simulink model "simple_relay_hysteresis"  (R2015a)
settings: Solver=ode45  StartTime=0.0  StopTime=tmax  RelTol=1e-3
values from neighbouring files (symbols this model uses):
  A = 5    [testing_simple_relay_hysteresis.m]
  b = 1    [testing_relay_plant_positive_feedback.m]    (also in testing_simple_relay_hysteresis.m = 1.5; testing_simple_relay_plant.m)
  d = 1    [testing_relay_plant_positive_feedback.m]    (also in testing_simple_relay_hysteresis.m = 2; testing_simple_relay_plant.m)
settings Model: Creator=ra428  LastModifiedBy=ra428

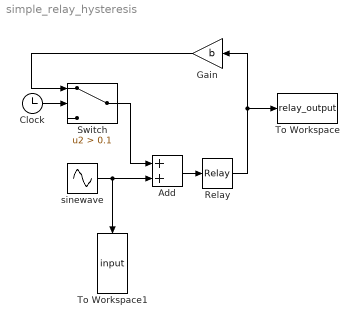
== system simple_relay_hysteresis ==
  Add : Sum
  Clock : Clock
  Gain : Gain  Gain=b
  Relay : Relay  OnSwitchValue=0  OffSwitchValue=0  OnOutputValue=d  OffOutputValue=-d
  Switch : Switch  Criteria=u2 > Threshold  Threshold=0.1
  To Workspace : ToWorkspace  VariableName=relay_output  SaveFormat=Timeseries  SampleTime=-1
  To Workspace1 : ToWorkspace  VariableName=input  SaveFormat=Timeseries  SampleTime=-1
  sinewave : Sin  Amplitude=A  Frequency=2  SampleTime=0
  wires:
  Relay/1 -> To Workspace/1, Gain/1
  Add/1 -> Relay/1
  Gain/1 -> Switch/1
  sinewave/1 -> Add/2, To Workspace1/1
  Switch/1 -> Add/1
  Clock/1 -> Switch/2
